simulink model "ReferenceGeneration"  (R2025a)
settings: Solver=FixedStepAuto  StartTime=0.0  StopTime=10.0  RelTol=1e-3
model mask{GridFrequency=GridFrequency, pUpperLimit=pUpperLimit, pLowerLimit=pLowerLimit, qUpperLimit=qUpperLimit, qLowerLimit=qLowerLimit}
  mask prompts: pUpperLimit "Maximum Value in pu"; pLowerLimit "Minimum Value in pu"; qUpperLimit "Maximum Value in pu"; qLowerLimit "Minimum Value in pu"
model workspace (MAT data in the model file):
  GridFrequency = 60
  pLowerLimit = 0
  pUpperLimit = 0
  qLowerLimit = 0
  qUpperLimit = 0
settings Model: ParameterArgumentNames=GridFrequency,pLowerLimit,pUpperLimit,qLowerLimit,qUpperLimit  Creator=skota  LastModifiedBy=skota
settings DataIOCC: SaveFormat=StructureWithTime  SaveOutput=off  SignalLogging=off  DSMLogging=off  SaveTime=off  ReturnWorkspaceOutputs=off
settings RTWCC: Toolchain=MinGW64 | CMake/gmake (64-bit Windows)  BuildConfiguration=Release  GPUComputeCapability=3.5

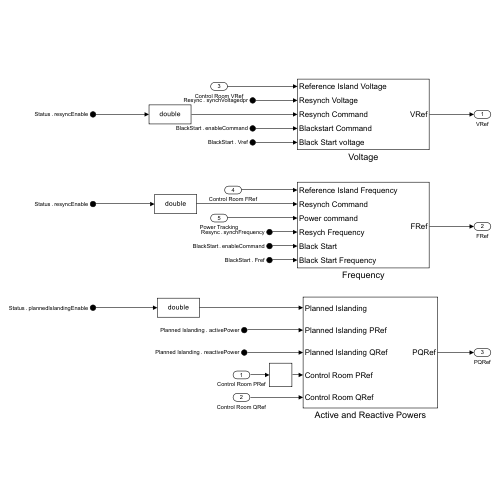
[thumbnail: Simulink's stored preview of the top-level diagram]
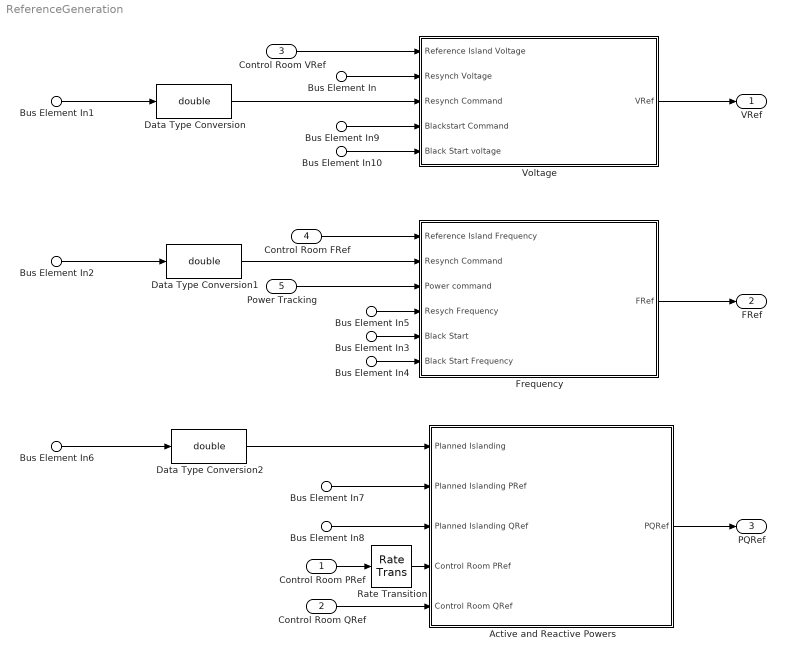
== system ReferenceGeneration ==
  Control Room PRef : Inport
  Control Room QRef : Inport  Port=2
  Control Room VRef : Inport  Port=3
  Control Room FRef : Inport  Port=4
  Power Tracking : Inport  Port=5
  Bus Element In : Inport  Port=6  PortName=Resync  Element=synchVoltagedpr
  Bus Element In5 : Inport  Port=6  PortName=Resync  Element=synchFrequency
  Bus Element In7 : Inport  Port=7  PortName=Planned Islanding  Element=activePower
  Bus Element In8 : Inport  Port=7  PortName=Planned Islanding  Element=reactivePower
  Bus Element In3 : Inport  Port=8  PortName=BlackStart  Element=enableCommand
  Bus Element In9 : Inport  Port=8  PortName=BlackStart  Element=enableCommand
  Bus Element In4 : Inport  Port=8  PortName=BlackStart  Element=Fref
  Bus Element In10 : Inport  Port=8  PortName=BlackStart  Element=Vref
  Bus Element In6 : Inport  Port=9  PortName=Status  Element=plannedIslandingEnable
  Bus Element In1 : Inport  Port=9  PortName=Status  Element=resyncEnable
  Bus Element In2 : Inport  Port=9  PortName=Status  Element=resyncEnable
  Active and Reactive Powers : Subsystem
  Data Type Conversion : DataTypeConversion  OutDataTypeStr=double  SaturateOnIntegerOverflow=off  RndMeth=Floor
  Data Type Conversion1 : DataTypeConversion  OutDataTypeStr=double  SaturateOnIntegerOverflow=off  RndMeth=Floor
  Data Type Conversion2 : DataTypeConversion  OutDataTypeStr=double  SaturateOnIntegerOverflow=off  RndMeth=Floor
  Frequency : Subsystem
  Rate Transition : RateTransition  OutPortSampleTime=1e-3
  Voltage : Subsystem
  VRef : Outport
  FRef : Outport  Port=2
  PQRef : Outport  Port=3
  wires:
  Bus Element In/1 -> Voltage/2(Resynch Voltage)
  Bus Element In4/1 -> Frequency/6(Black Start Frequency)
  Frequency/1(FRef) -> FRef/1
  Active and Reactive Powers/1(PQRef) -> PQRef/1
  Bus Element In10/1 -> Voltage/5(Black Start voltage)
  Bus Element In5/1 -> Frequency/4(Resych Frequency)
  Voltage/1(VRef) -> VRef/1
  Bus Element In8/1 -> Active and Reactive Powers/3(Planned Islanding QRef)
  Bus Element In9/1 -> Voltage/4(Blackstart Command)
  Bus Element In7/1 -> Active and Reactive Powers/2(Planned Islanding PRef)
  Bus Element In3/1 -> Frequency/5(Black Start)
  Data Type Conversion/1 -> Voltage/3(Resynch Command)
  Data Type Conversion1/1 -> Frequency/2(Resynch Command)
  Data Type Conversion2/1 -> Active and Reactive Powers/1(Planned Islanding)
  Power Tracking/1 -> Frequency/3(Power command)
  Control Room VRef/1 -> Voltage/1(Reference Island Voltage)
  Control Room FRef/1 -> Frequency/1(Reference Island Frequency)
  Control Room QRef/1 -> Active and Reactive Powers/5(Control Room QRef)
  Bus Element In1/1 -> Data Type Conversion/1
  Bus Element In2/1 -> Data Type Conversion1/1
  Bus Element In6/1 -> Data Type Conversion2/1
  Control Room PRef/1 -> Rate Transition/1
  Rate Transition/1 -> Active and Reactive Powers/4(Control Room PRef)

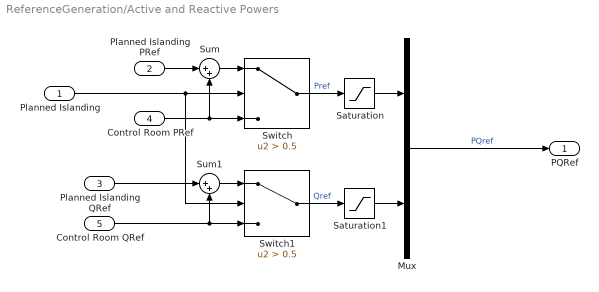
== system ReferenceGeneration/Active and Reactive Powers ==
  Planned Islanding : Inport
  Planned Islanding PRef : Inport  Port=2
  Planned Islanding QRef : Inport  Port=3
  Control Room PRef : Inport  Port=4
  Control Room QRef : Inport  Port=5
  Mux : Mux  Inputs=2
  Saturation : Saturate  UpperLimit=pUpperLimit  LowerLimit=pLowerLimit
  Saturation1 : Saturate  UpperLimit=qUpperLimit  LowerLimit=qLowerLimit
  Sum : Sum  Inputs=|++
  Sum1 : Sum  Inputs=|++
  Switch : Switch  Criteria=u2 > Threshold  Threshold=0.5  SaturateOnIntegerOverflow=off  InputSameDT=off
  Switch1 : Switch  Criteria=u2 > Threshold  Threshold=0.5  SaturateOnIntegerOverflow=off  InputSameDT=off
  PQRef : Outport
  wires:
  Saturation1/1 -> Mux/2
  Saturation/1 -> Mux/1
  Switch/1 -> Saturation/1  "Pref"
  Planned Islanding PRef/1 -> Sum/1
  Planned Islanding QRef/1 -> Sum1/1
  Mux/1 -> PQRef/1  "PQref"
  Sum/1 -> Switch/1
  Switch1/1 -> Saturation1/1  "Qref"
  Sum1/1 -> Switch1/1
  Control Room PRef/1 -> Switch/3, Sum/2
  Control Room QRef/1 -> Sum1/2, Switch1/3
  Planned Islanding/1 -> Switch1/2, Switch/2

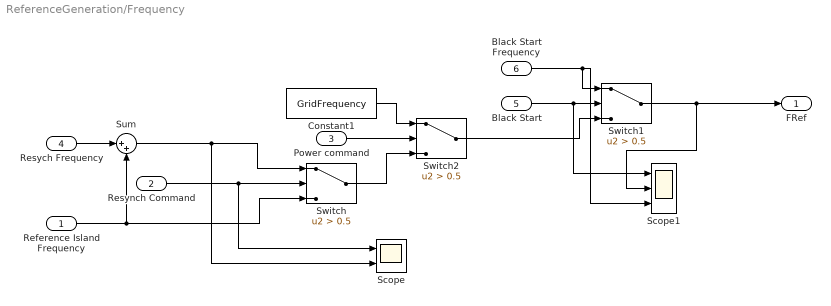
== system ReferenceGeneration/Frequency ==
  Reference Island Frequency : Inport
  Resynch Command : Inport  Port=2
  Power command : Inport  Port=3
  Resych Frequency : Inport  Port=4
  Black Start : Inport  Port=5
  Black Start Frequency : Inport  Port=6
  Constant1 : Constant  Value=GridFrequency
  Scope : Scope  NumInputPorts=2
      settings: DataLoggingVariableName=ScopeData2
  Scope1 : Scope  NumInputPorts=3
      settings: DataLoggingVariableName=ScopeData3
  Sum : Sum  Inputs=|++
  Switch : Switch  Criteria=u2 > Threshold  Threshold=0.5  SaturateOnIntegerOverflow=off  InputSameDT=off
  Switch1 : Switch  Criteria=u2 > Threshold  Threshold=0.5  SaturateOnIntegerOverflow=off  InputSameDT=off
  Switch2 : Switch  Criteria=u2 > Threshold  Threshold=0.5  SaturateOnIntegerOverflow=off  InputSameDT=off
  FRef : Outport
  wires:
  Switch2/1 -> Switch1/3
  Resych Frequency/1 -> Sum/1
  Black Start Frequency/1 -> Scope1/3, Switch1/1
  Black Start/1 -> Scope1/1, Switch1/2
  Power command/1 -> Switch2/2
  Reference Island Frequency/1 -> Sum/2, Switch/3
  Sum/1 -> Scope/2, Switch/1
  Constant1/1 -> Switch2/1
  Switch/1 -> Switch2/3
  Switch1/1 -> Scope1/2, FRef/1
  Resynch Command/1 -> Scope/1, Switch/2

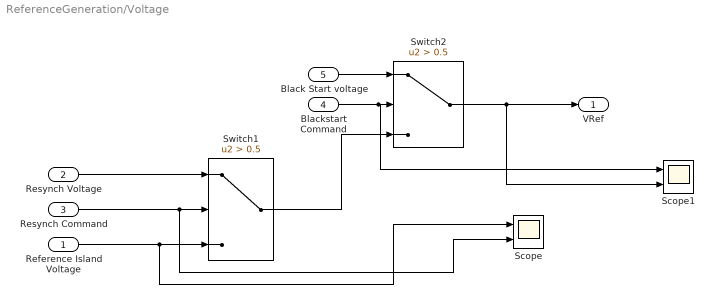
== system ReferenceGeneration/Voltage ==
  Reference Island Voltage : Inport
  Resynch Voltage : Inport  Port=2
  Resynch Command : Inport  Port=3
  Blackstart Command : Inport  Port=4
  Black Start voltage : Inport  Port=5
  Scope : Scope  NumInputPorts=2
  Scope1 : Scope  NumInputPorts=2
  Switch1 : Switch  Criteria=u2 > Threshold  Threshold=0.5  SaturateOnIntegerOverflow=off  InputSameDT=off
  Switch2 : Switch  Criteria=u2 > Threshold  Threshold=0.5  SaturateOnIntegerOverflow=off  InputSameDT=off
  VRef : Outport
  wires:
  Switch2/1 -> Scope1/2, VRef/1
  Switch1/1 -> Switch2/3
  Reference Island Voltage/1 -> Scope/1, Switch1/3
  Blackstart Command/1 -> Scope1/1, Switch2/2
  Black Start voltage/1 -> Switch2/1
  Resynch Voltage/1 -> Switch1/1
  Resynch Command/1 -> Scope/2, Switch1/2
